simulink model "Scenario1"  (R2023a)
settings: Solver=VariableStepAuto  StartTime=0.0  StopTime=30  RelTol=1e-3
libraries: simulink x1
settings Model: Creator=Νίκος  LastModifiedBy=Νίκος

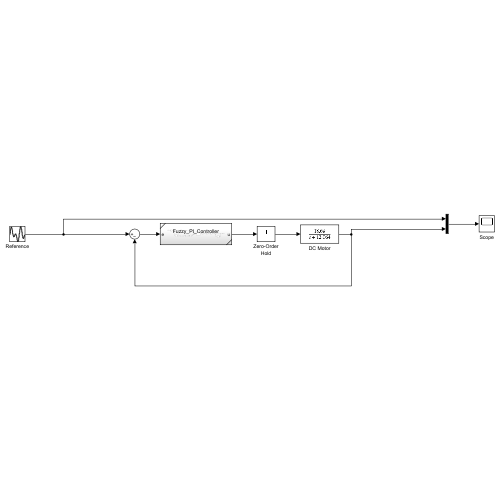
[thumbnail: Simulink's stored preview of the top-level diagram]
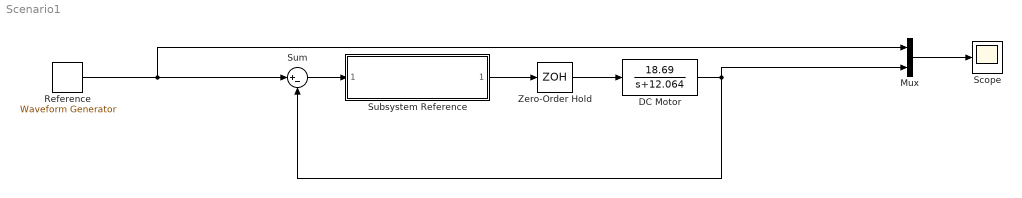
== system Scenario1 ==
  DC Motor : TransferFcn  Numerator=[18.69]  Denominator=[1 12.064]
  Mux : Mux  Inputs=2
  Reference : simulink/Sources/Waveform Generator  OutMin=[]  OutMax=[]  OutDataTypeStr=double  SelectedSignal=1  Signals=step(0,0,150) - step(10,0,50) + step(20,0,50)  BlockNames=MultiportSwitch_c1f955a0ecf14bb  SampleTime=0.01
  Scope : Scope
  Subsystem Reference : Subsystem  ReferencedSubsystem=Fuzzy_PI_Controller
  Sum : Sum  Inputs=|+-
  Zero-Order Hold : ZeroOrderHold  SampleTime=-1
  wires:
  Reference/1 -> Mux/1, Sum/1
  Sum/1 -> Subsystem Reference/1
  Zero-Order Hold/1 -> DC Motor/1
  DC Motor/1 -> Mux/2, Sum/2
  Subsystem Reference/1 -> Zero-Order Hold/1
  Mux/1 -> Scope/1
